simulink model "powertrain_model_simulink"  (R2023b)
settings: Solver=VariableStepAuto  StartTime=0.0  StopTime=20  RelTol=1e-3
undefined symbols (not defined in the file or in its folder): ts_equivalent_resistance
libraries: nesl_utility x9, fl_lib x7, ee_lib x7, simulink x1, batt_lib x1
settings Model: Creator=bglen  LastModifiedBy=bglen

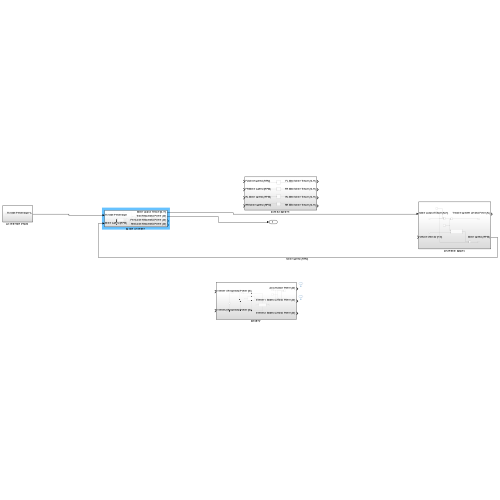
[thumbnail: Simulink's stored preview of the top-level diagram]
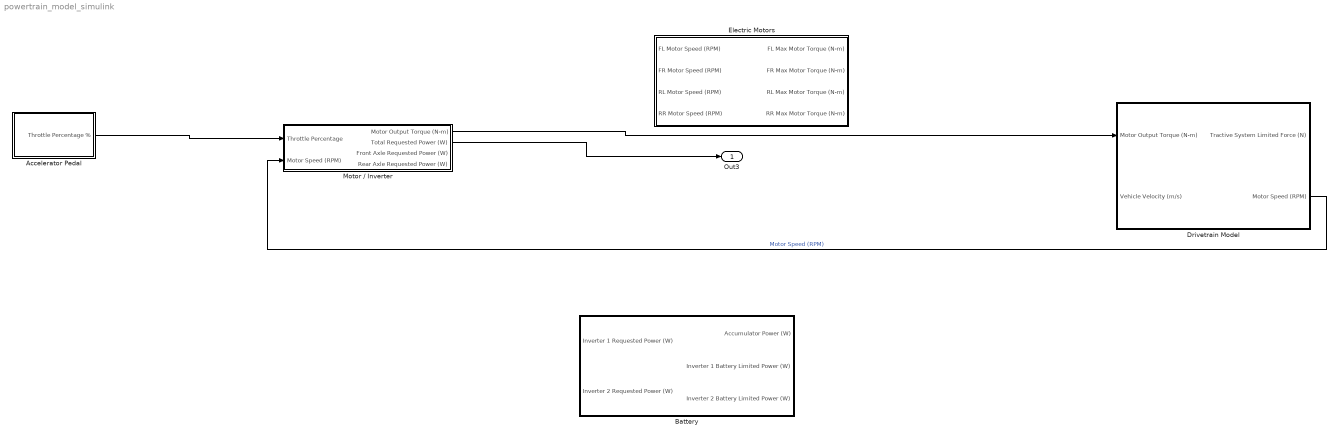
== system powertrain_model_simulink ==
  Accelerator Pedal : Subsystem
  Battery : Subsystem
  Drivetrain Model : Subsystem
  Electric Motors : Subsystem
  Motor / Inverter : Subsystem
  Out3 : Outport
  wires:
  Motor / Inverter/1(Motor Output Torque (N-m)) -> Drivetrain Model/1(Motor Output Torque (N-m))
  Motor / Inverter/2(Total Requested Power (W)) -> Out3/1
  Accelerator Pedal/1(Throttle Percentage %) -> Motor / Inverter/1(Throttle Percentage)
  Drivetrain Model/2(Motor Speed (RPM)) -> Motor / Inverter/2(Motor Speed (RPM))  "Motor Speed (RPM)"

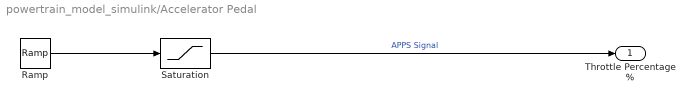
== system powertrain_model_simulink/Accelerator Pedal ==
  Ramp : simulink/Sources/Ramp  slope=4  start=0  InitialOutput=0
  Saturation : Saturate  UpperLimit=1  LowerLimit=0
  Throttle Percentage % : Outport
  wires:
  Saturation/1 -> Throttle Percentage %/1  "APPS Signal"
  Ramp/1 -> Saturation/1

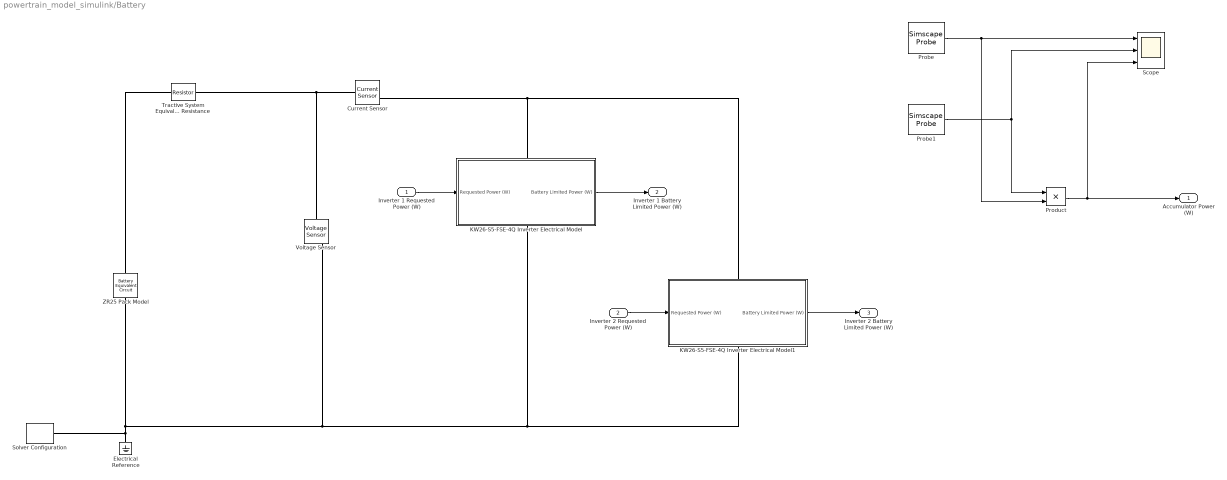
== system powertrain_model_simulink/Battery ==
  Inverter 1 Requested Power (W) : Inport
  Inverter 2 Requested Power (W) : Inport  Port=2
  Current Sensor : fl_lib/Electrical/Electrical Sensors/Current Sensor
  Electrical Reference : fl_lib/Electrical/Electrical Elements/Electrical Reference
  KW26-S5-FSE-4Q Inverter Electrical Model : Subsystem
      settings: PortSchema="{\"entries\":[{\"content\":{\"sides\":[{\"content\":{\"connectorIds\":[\"In1\"]},\"type\":\"ConnectorPlacement.EquallySpacedRectSide\",\"uuid\":\"23f200cd-6174-4ea5-b281-640ad05ed590\"},{\"content\":{\"connectorIds\":[\"Out1\"],\"side\":\"RIGHT\"},\"type\":\"ConnectorPlacement.EquallySpacedRectSide\",\"uuid\":\"19e54f00-a657-433d-b717-823657cd0153\"},{\"content\":{\"connectorIds\":[\"LConn1\"],\"side\":\"TOP\"},\"type\":\"ConnectorPlacement.EquallySpacedRectSide\",\"uuid\":\"a44b7635-6f3a-41c2-8d23-941c3ed86804\"},{\"content\":{\"connectorIds\":[\"RConn1\"],\"side\":\"BOTTOM\"},\"type\":\"ConnectorPlacement.EquallySpacedRectSide\",\"uuid\":\"02d96f81-f414-45e4-b3a2-9210237ffb13\"}]},\"type\":\"ConnectorPlacement.EquallySpacedConnector\",\"uuid\":\"152a73da-5f7e-4c02-a782-729b53bb1c10\"}],\"packageUris\":[\"http://schema.mathworks.com/mf0/Connector/R2020b\"],\"version\":\"1.0\"}"
  KW26-S5-FSE-4Q Inverter Electrical Model1 : Subsystem
      settings: PortSchema="{\"entries\":[{\"content\":{\"sides\":[{\"content\":{\"connectorIds\":[\"In1\"]},\"type\":\"ConnectorPlacement.EquallySpacedRectSide\",\"uuid\":\"23f200cd-6174-4ea5-b281-640ad05ed590\"},{\"content\":{\"connectorIds\":[\"Out1\"],\"side\":\"RIGHT\"},\"type\":\"ConnectorPlacement.EquallySpacedRectSide\",\"uuid\":\"19e54f00-a657-433d-b717-823657cd0153\"},{\"content\":{\"connectorIds\":[\"LConn1\"],\"side\":\"TOP\"},\"type\":\"ConnectorPlacement.EquallySpacedRectSide\",\"uuid\":\"a44b7635-6f3a-41c2-8d23-941c3ed86804\"},{\"content\":{\"connectorIds\":[\"RConn1\"],\"side\":\"BOTTOM\"},\"type\":\"ConnectorPlacement.EquallySpacedRectSide\",\"uuid\":\"02d96f81-f414-45e4-b3a2-9210237ffb13\"}]},\"type\":\"ConnectorPlacement.EquallySpacedConnector\",\"uuid\":\"152a73da-5f7e-4c02-a782-729b53bb1c10\"}],\"packageUris\":[\"http://schema.mathworks.com/mf0/Connector/R2020b\"],\"version\":\"1.0\"}"
  Probe : SimscapeProbe  BoundBlock=271  Variables={V}
  Probe1 : SimscapeProbe  BoundBlock=272  Variables={I}
  Product : Product
  Scope : Scope  NumInputPorts=3
  Solver Configuration : nesl_utility/Solver Configuration  PhysicalDomain=network_engine_domain  SubClassName=solver  LeftPortType=input  RightPortType=generic  Tones=[]  Harmonics=[]  SimulateNoise=off  Profile=off  UseLocalSampling=off  EnableSwitchedLinearOptims=on  FrequencyDomain=off  UseCCode=off  RelTol=0.001  AbsTol=0.001  MinStep=1e-09  ToWorkspace=off  RevertToSquareIcSolve=off  NumHomotopyIterations=100  PhasorMode=off  PhasorModeNumHarmonics=1  ConsistencySolver=NEWTON_XTOL_AFTER_FTOL  IndexReductionMethod=DerivativeReplacement  DoDC=off  ResidualTolerance=1e-09  ConsistencyTolSource=GLOBAL  ConsistencyAbsTol=0.001  ConsistencyRelTol=0.001  ConsistencyTolFactor=0.001  UseLocalSolver=off  LocalSolverChoice=NE_BACKWARD_EULER_ADVANCER  ResolveIndetEquations=on  FunctionEvalNumThread=1  LocalSolverSampleTime=0.001  DoFixedCost=off  MaxNonlinIter=3  MaxModeIter=2  ComputeImpulses=off  ImpulseIterations=2  LinearAlgebra=auto  LinearAlgebraNumThread=0  EquationFormulation=NE_TIME_EF  DelaysMemoryBudget=1024  AutomaticFiltering=on  FilteringTimeConstant=0.001  PartitionStorageMethod=AS_NEEDED  PartitionMemoryBudget=1024  PartitionMethod=ROBUST  MultibodyUseLocalSolver=off  MultibodyLocalSolverChoice=ODE1  MultibodyLocalSolverSampleTime=0.001
  Tractive System Equivalent Resistance : ee_lib/Passive/Resistor  R=ts_equivalent_resistance Ohm  enable_R_tol=ee.enum.toleranceApplication.none  R_tol=5  tol_distribution=ee.enum.toleranceDistribution.uniform  nSigma=4  enable_operating_limits=ee.enum.enable.no  operating_limit_action=ee.enum.passive.reportOpLim.warn  power_rating=1 W  max_working_voltage=100 V  enable_faults=ee.enum.enable.no  fault_action=simscape.enum.assert.action.none  R_faulted=inf Ohm  fault_trigger=ee.enum.faults.faultTrigger.temporal  t_fault=1 s  max_permissible_current=1 A  t_fail_on_current=1 s  noise_mode=ee.enum.sources.noise.Disabled  Tdevice=25 degC  sample_time=1e-3 s  repeatability=ee.enum.ic.repeatability.notRepeatable  user_seed=0  auto_seed=3499211588  faulted_specify=off  faulted_priority=None  faulted=0  power_derating_T1=70 degC  power_derating_T2=155 degC  operating_temperature_range_vec=[-50, 150] degC  alpha=3.93e-3 1/K  Tmeas=25 degC  thermal_mass=100 J/K  temperature_specify=off  temperature_priority=High  temperature=298.15 K  temperature_nominal_specify=off  temperature_nominal_unit=K  temperature_nominal_value=1
  Voltage Sensor : fl_lib/Electrical/Electrical Sensors/Voltage Sensor
  ZR25 Pack Model : batt_lib/Cells/Battery Equivalent Circuit  BatteryCapacity=pack_nominal_capacity A*hr  ThermalModel=simscape.battery.enum.cells.BatteryThermalModel.ConstantTemperature  ExtrapolationMethod=simscape.enum.extrapolation.nearest  EnableFaultExotherm=false  TriggerTemperature=350 K  SOCBreakpoints=pack_SOC  TemperatureBreakpoints=pack_temps degC  OpenCircuitVoltage=[3.5057, 3.566, 3.6337, 3.7127, 3.9259, 4.0777, 4.1928] V  OpenCircuitVoltageThermal=pack_OCV V  VoltageRange=[0, inf] V  HysteresisModel=simscape.battery.enum.cells.HysteresisModel.none  MaximumHysteresisVoltage=[0, 0, 0, 0, 0, 0, 0] V  InstantaneousHysteresisVoltage=[0, 0, 0, 0, 0, 0, 0] V  HysteresisRate=0.1  MaximumHysteresisVoltageThermal=[0, 0, 0; 0, 0, 0; 0, 0, 0; 0, 0, 0; 0, 0, 0; 0, 0, 0; 0, 0, 0] V  InstantaneousHysteresisVoltageThermal=[0, 0, 0; 0, 0, 0; 0, 0, 0; 0, 0, 0; 0, 0, 0; 0, 0, 0; 0, 0, 0] V  HysteresisRateThermal=0.1  ResistanceSOCBreakpoints=pack_SOC  ResistanceTemperatureBreakpoints=pack_temps degC  CurrentDirectionality=simscape.battery.enum.cells.BatteryEnable.Disabled  R0=[.0085, .0085, .0087, .0082, .0083, .0085, .0085] Ohm  R0Thermal=pack_DC_IR Ohm  DischargeR0=[.0085, .0085, .0087, .0082, .0083, .0085, .0085] Ohm  ChargeR0=[.0085, .0085, .0087, .0082, .0083, .0085, .0085] Ohm  ChargeR0Thermal=[.0117, .0085, .009; .011, .0085, .009; .0114, .0087, .0092; .0107, .0082, .0088; .0107, .0083, .0091; .0113, .0085, .0089; .0116, .0085, .0089] Ohm  DischargeR0Thermal=[.0117, .0085, .009; .011, .0085, .009; .0114, .0087, .0092; .0107, .0082, .0088; .0107, .0083, .0091; .0113, .0085, .0089; .0116, .0085, .0089] Ohm  SelfDischargeResistor=simscape.battery.enum.cells.BatteryEnable.Disabled  SelfDischargeR=7e3 Ohm  SelfDischargeRThermal=[8000, 7000, 6000] Ohm  RCPairs=simscape.battery.enum.cells.RCPairs.noDynamics  R1=[.0029, .0024, .0026, .0016, .0023, .0018, .0017] Ohm  Tau1=[36, 45, 105, 29, 77, 33, 39] s  R2=[.0029, .0024, .0026, .0016, .0023, .0018, .0017] Ohm  Tau2=[36, 45, 105, 29, 77, 33, 39] s  R3=[.0029, .0024, .0026, .0016, .0023, .0018, .0017] Ohm  Tau3=[36, 45, 105, 29, 77, 33, 39] s  DischargeR1=[.0029, .0024, .0026, .0016, .0023, .0018, .0017] Ohm  DischargeTau1=[36, 45, 105, 29, 77, 33, 39] s  ChargeR1=[.0029, .0024, .0026, .0016, .0023, .0018, .0017] Ohm  ChargeTau1=[36, 45, 105, 29, 77, 33, 39] s  DischargeR2=[.0029, .0024, .0026, .0016, .0023, .0018, .0017] Ohm  DischargeTau2=[36, 45, 105, 29, 77, 33, 39] s  ChargeR2=[.0029, .0024, .0026, .0016, .0023, .0018, .0017] Ohm  ChargeTau2=[36, 45, 105, 29, 77, 33, 39] s  DischargeR3=[.0029, .0024, .0026, .0016, .0023, .0018, .0017] Ohm  DischargeTau3=[36, 45, 105, 29, 77, 33, 39] s  ChargeR3=[.0029, .0024, .0026, .0016, .0023, .0018, .0017] Ohm  ChargeTau3=[36, 45, 105, 29, 77, 33, 39] s  R1Thermal=[.0109, .0029, .0013; .0069, .0024, .0012; .0047, .0026, .0013; .0034, .0016, .001; .0033, .0023, .0014; .0033, .0018, .0011; .0028, .0017, .0011] Ohm  Tau1Thermal=[20, 36, 39; 31, 45, 39; 109, 105, 61; 36, 29, 26; 59, 77, 67; 40, 33, 29; 25, 39, 33] s  R2Thermal=[.0109, .0029, .0013; .0069, .0024, .0012; .0047, .0026, .0013; .0034, .0016, .001; .0033, .0023, .0014; .0033, .0018, .0011; .0028, .0017, .0011] Ohm  Tau2Thermal=[20, 36, 39; 31, 45, 39; 109, 105, 61; 36, 29, 26; 59, 77, 67; 40, 33, 29; 25, 39, 33] s  R3Thermal=[.0109, .0029, .0013; .0069, .0024, .0012; .0047, .0026, .0013; .0034, .0016, .001; .0033, .0023, .0014; .0033, .0018, .0011; .0028, .0017, .0011] Ohm  Tau3Thermal=[20, 36, 39; 31, 45, 39; 109, 105, 61; 36, 29, 26; 59, 77, 67; 40, 33, 29; 25, 39, 33] s  DischargeR1Thermal=[.0109, .0029, .0013; .0069, .0024, .0012; .0047, .0026, .0013; .0034, .0016, .001; .0033, .0023, .0014; .0033, .0018, .0011; .0028, .0017, .0011] Ohm  DischargeTau1Thermal=[20, 36, 39; 31, 45, 39; 109, 105, 61; 36, 29, 26; 59, 77, 67; 40, 33, 29; 25, 39, 33] s  ChargeR1Thermal=[.0109, .0029, .0013; .0069, .0024, .0012; .0047, .0026, .0013; .0034, .0016, .001; .0033, .0023, .0014; .0033, .0018, .0011; .0028, .0017, .0011] Ohm  ChargeTau1Thermal=[20, 36, 39; 31, 45, 39; 109, 105, 61; 36, 29, 26; 59, 77, 67; 40, 33, 29; 25, 39, 33] s  DischargeR2Thermal=[.0109, .0029, .0013; .0069, .0024, .0012; .0047, .0026, .0013; .0034, .0016, .001; .0033, .0023, .0014; .0033, .0018, .0011; .0028, .0017, .0011] Ohm  DischargeTau2Thermal=[20, 36, 39; 31, 45, 39; 109, 105, 61; 36, 29, 26; 59, 77, 67; 40, 33, 29; 25, 39, 33] s  ChargeR2Thermal=[.0109, .0029, .0013; .0069, .0024, .0012; .0047, .0026, .0013; .0034, .0016, .001; .0033, .0023, .0014; .0033, .0018, .0011; .0028, .0017, .0011] Ohm  ChargeTau2Thermal=[20, 36, 39; 31, 45, 39; 109, 105, 61; 36, 29, 26; 59, 77, 67; 40, 33, 29; 25, 39, 33] s  DischargeR3Thermal=[.0109, .0029, .0013; .0069, .0024, .0012; .0047, .0026, .0013; .0034, .0016, .001; .0033, .0023, .0014; .0033, .0018, .0011; .0028, .0017, .0011] Ohm  DischargeTau3Thermal=[20, 36, 39; 31, 45, 39; 109, 105, 61; 36, 29, 26; 59, 77, 67; 40, 33, 29; 25, 39, 33] s  ChargeR3Thermal=[.0109, .0029, .0013; .0069, .0024, .0012; .0047, .0026, .0013; .0034, .0016, .001; .0033, .0023, .0014; .0033, .0018, .0011; .0028, .0017, .0011] Ohm  ChargeTau3Thermal=[20, 36, 39; 31, 45, 39; 109, 105, 61; 36, 29, 26; 59, 77, 67; 40, 33, 29; 25, 39, 33] s  CyclingAgingMethod=simscape.battery.enum.cells.CyclingAgingMethod.disabled  NumDisCycles=100  OCVChange=0  R0Change=0  CapacityChange=0  SelfDischargeRChange=0  R1Change=0  R2Change=0  R3Change=0  NumDisCyclesBreakpoints=[0, 100, 200, 300]  AgingTemperatureBreakpoints=[298.15, 323.15] K  OCVChangeVec=[0, 0, 0, 0]  R0ChangeVec=[0, 0, 0, 0]  CapacityChangeVec=[0, 0, 0, 0]  SelfDischargeRChangeVec=[0, 0, 0, 0]  R1ChangeVec=[0, 0, 0, 0]  R2ChangeVec=[0, 0, 0, 0]  R3ChangeVec=[0, 0, 0, 0]  OCVChangeThermal=[0, 0; 0, 0; 0, 0; 0, 0]  R0ChangeThermal=[0, 0; 0, 0; 0, 0; 0, 0]  CapacityChangeThermal=[0, 0; 0, 0; 0, 0; 0, 0]  SelfDischargeRChangeThermal=[0, 0; 0, 0; 0, 0; 0, 0]  R1ChangeThermal=[0, 0; 0, 0; 0, 0; 0, 0]  R2ChangeThermal=[0, 0; 0, 0; 0, 0; 0, 0]  R3ChangeThermal=[0, 0; 0, 0; 0, 0; 0, 0]  CalendarAgeResistance=simscape.battery.enum.cells.BatteryEnable.Disabled  CalendarAgeCapacity=simscape.battery.enum.cells.BatteryEnable.Disabled  CalendarAgingMethod=simscape.battery.enum.cells.CalendarAgingMethod.equation  StorageVariable=simscape.battery.enum.cells.StorageVariable.OCV  OCVDuringStorage=0.9  SOCDuringStorage=0.6  StorageTimeIntervals=[0] d  StorageTemperatures=[273] K  ResistanceScalingOCV=2.2134e6  ResistanceScalingOCVOffset=1.632e6  ResistanceExponentialIncrease=0.515833569 V  ResistanceTimeExponent=0.75  ResistanceAgeTemperatureBreakpoints=[273.15, 298.15, 323.15] K  ResistanceAgeTimeBreakpoints=[0, 90, 180, 270] d  PercentResistanceChange=[0, 0, 0]  ResistanceTimeBreakpoints=100 d  PercentResistanceChangeThermal=[0, 0, 0; 0, 0, 0; 0, 0, 0; 0, 0, 0]  CapacityScalingOCV=1.5097e07  CapacityScalingOCVOffset=8.3625e06  CapacityExponentialIncrease=0.6011 V  CapacityTimeExponent=0.75  CapacityAgeTemperatureBreakpoints=[273.15, 298.15, 323.15] K  CapacityAgeTimeBreakpoints=[0, 90, 180, 270] d  PercentCapacityChange=[0, 0, 0]  CapacityTimeBreakpoints=100 d  PercentCapacityChangeThermal=[0, 0, 0; 0, 0, 0; 0, 0, 0; 0, 0, 0]  SimulationTemperature=298.15 degC  BatteryThermalMass=100 J/K  ReversibleHeatModel=simscape.battery.enum.cells.ReversibleHeatModel.Disabled  EntropicCoefficient=[0, 0, 0, 0, 0, 0, 0] mV/K  AddedResistance=1e5 Ohm  ShortedResistance=1e-6 Ohm  ExothermModel=simscape.battery.enum.cells.ExothermModel.analytical  TabulateWithSOC=false  SOCvecExotherm=[0, .5, 1]  CurrInterruptTempSOC=[420, 420, 420] K  TotalHeatOfReactionSOC=[23000, 23000, 23000] J  CurrentInterruptTemperature=420 K  TotalHeatOfReaction=23e3 J  ExothermOnsetTemperature=350 K  ExothermOnsetTempSOC=[350, 350, 350] K  OnsetTempRate=0.02 K/min  ActivationEnergy=160e3 J/mol  ActivationEnergySOC=[160000, 160000, 160000] J/mol  ReactionOrder=1  ReactionOrderSOC=[1, 1, 1]  TemperaturesFromARC=[323, 373, 423, 438, 463, 483, 513, 543, 545, 547, 549, 551, 553, 573, 623, 773, 923, 943, 1003, 1063, 1113, 1123, 1133, 1153, 1173] K  TemperatureRatesFromARC=[.0001, .001, .025, .2, .4, .6, 1.1, 1.3, 1.9, 3, 5, 11.6, 183.3, 191.6, 200, 208.3, 200, 175, 8.33, 1.33, .33, .2, .13, .0017, .00017] K/s  TempRateVecARCSOC=repmat([.0001, .001, .025, .2, .4, .6, 1.1, 1.3, 1.9, 3, 5, 11.6, 183.3, 191.6, 200, 208.3, 200, 175, 8.33, 1.33, .33, .2, .13, .0017, .00017]', 1, 3) K/s  PercentThermalMassVented=40  PercentThermalMassVentedSOC=[40, 40, 40]  EnableFaultAddRes=false  EnableFaultShort=false  faultTriggerType=simscape.fault.triggertype.external  stateOfCharge_specify=on  stateOfCharge_priority=High  stateOfCharge=1  stateOfCharge_nominal_specify=off  stateOfCharge_nominal_unit=1  stateOfCharge_nominal_value=1  numCycles_specify=off  numCycles_priority=High  numCycles=0  numCycles_nominal_specify=off  numCycles_nominal_unit=1  numCycles_nominal_value=1  batteryVoltage_specify=off  batteryVoltage_priority=None  batteryVoltage=0 V  batteryVoltage_nominal_specify=off  batteryVoltage_nominal_unit=V  batteryVoltage_nominal_value=3.73  batteryCurrent_specify=off  batteryCurrent_priority=None  batteryCurrent=0 A  batteryCurrent_nominal_specify=off  batteryCurrent_nominal_unit=A  batteryCurrent_nominal_value=1  batteryTemperature_specify=off  batteryTemperature_priority=High  batteryTemperature=298.15 K  batteryTemperature_nominal_specify=off  batteryTemperature_nominal_unit=K  batteryTemperature_nominal_value=1  hysteresisState_specify=off  hysteresisState_priority=High  hysteresisState=0  hysteresisState_nominal_specify=off  hysteresisState_nominal_unit=1  hysteresisState_nominal_value=1  isExothermFaulted_specify=off  isExothermFaulted_priority=None  isExothermFaulted=0  isExothermFaulted_nominal_specify=off  isExothermFaulted_nominal_unit=1  isExothermFaulted_nominal_value=1  isCurrentInterruptionTempExceeded_specify=off  isCurrentInterruptionTempExceeded_priority=None  isCurrentInterruptionTempExceeded=0  isCurrentInterruptionTempExceeded_nominal_specify=off  isCurrentInterruptionTempExceeded_nominal_unit=1  isCurrentInterruptionTempExceeded_nominal_value=1  reactionHeatRate_specify=off  reactionHeatRate_priority=None  reactionHeatRate=0 W  reactionHeatRate_nominal_specify=off  reactionHeatRate_nominal_unit=W  reactionHeatRate_nominal_value=1  reactionExtent_specify=off  reactionExtent_priority=None  reactionExtent=0  reactionExtent_nominal_specify=off  reactionExtent_nominal_unit=1  reactionExtent_nominal_value=1
      settings: InternalSimscapePortConfiguration="{\"Bottom\":[],\"Left\":[{\"id\":\"p\",\"label\":\"+\",\"type\":\"foundation.electrical.electrical\"}],\"Right\":[{\"id\":\"n\",\"label\":\"-\",\"type\":\"foundation.electrical.electrical\"}],\"Top\":[]}"
  Accumulator Power (W) : Outport
  Inverter 1 Battery Limited Power (W) : Outport  Port=2
  Inverter 2 Battery Limited Power (W) : Outport  Port=3
  wires:
  Probe/1 -> Scope/1, Product/2
  Probe1/1 -> Scope/2, Product/1
  Product/1 -> Accumulator Power (W)/1, Scope/3
  Inverter 1 Requested Power (W)/1 -> KW26-S5-FSE-4Q Inverter Electrical Model/1(Requested Power (W))
  KW26-S5-FSE-4Q Inverter Electrical Model/1(Battery Limited Power (W)) -> Inverter 1 Battery Limited Power (W)/1
  KW26-S5-FSE-4Q Inverter Electrical Model1/1(Battery Limited Power (W)) -> Inverter 2 Battery Limited Power (W)/1
  Inverter 2 Requested Power (W)/1 -> KW26-S5-FSE-4Q Inverter Electrical Model1/1(Requested Power (W))
  connections:
  Electrical Reference/LConn1 -- KW26-S5-FSE-4Q Inverter Electrical Model1/RConn1 -- KW26-S5-FSE-4Q Inverter Electrical Model/RConn1 -- Voltage Sensor/RConn2 -- ZR25 Pack Model/RConn1 -- Solver Configuration/RConn1
  Tractive System Equivalent Resistance/RConn1 -- Current Sensor/LConn1 -- Voltage Sensor/LConn1
  Current Sensor/RConn2 -- KW26-S5-FSE-4Q Inverter Electrical Model1/LConn1 -- KW26-S5-FSE-4Q Inverter Electrical Model/LConn1
  Tractive System Equivalent Resistance/LConn1 -- ZR25 Pack Model/LConn1

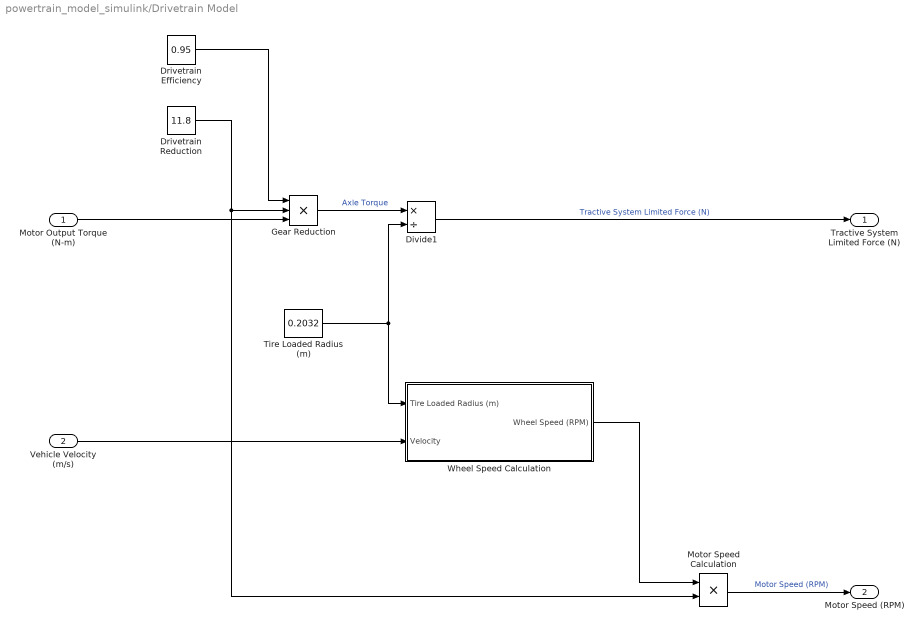
== system powertrain_model_simulink/Drivetrain Model ==
  Motor Output Torque (N-m) : Inport
  Vehicle Velocity (m/s) : Inport  Port=2
  "  Motor Speed Calculation" : Product
  Divide1 : Product  Inputs=*/
  Drivetrain Efficiency : Constant  Value=0.95
  Drivetrain Reduction : Constant  Value=11.8
  Gear Reduction : Product  Inputs=3
  Tire Loaded Radius (m) : Constant  Value=0.2032
  Wheel Speed Calculation : Subsystem
  Tractive System Limited Force (N) : Outport
  Motor Speed (RPM) : Outport  Port=2
  wires:
  Divide1/1 -> Tractive System Limited Force (N)/1  "Tractive System Limited Force (N)"
  Tire Loaded Radius (m)/1 -> Wheel Speed Calculation/1(Tire Loaded Radius (m)), Divide1/2
  Gear Reduction/1 -> Divide1/1  "Axle Torque"
  Motor Output Torque (N-m)/1 -> Gear Reduction/3
  Drivetrain Efficiency/1 -> Gear Reduction/1
  Drivetrain Reduction/1 -> "  Motor Speed Calculation"/2, Gear Reduction/2
  Vehicle Velocity (m/s)/1 -> Wheel Speed Calculation/2(Velocity)
  Wheel Speed Calculation/1(Wheel Speed (RPM)) -> "  Motor Speed Calculation"/1
  "  Motor Speed Calculation"/1 -> Motor Speed (RPM)/1  "Motor Speed (RPM)"

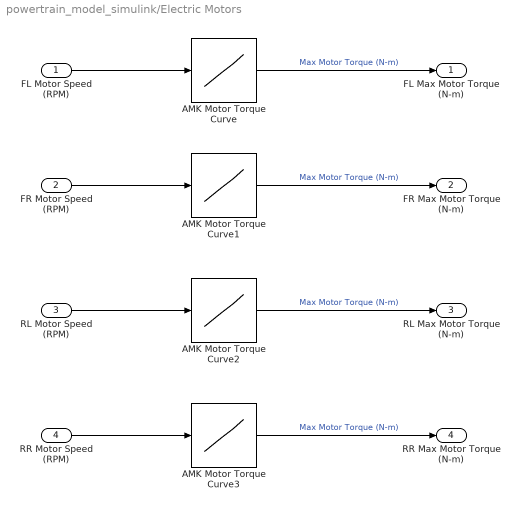
== system powertrain_model_simulink/Electric Motors ==
  FL Motor Speed (RPM) : Inport
  FR Motor Speed (RPM) : Inport  Port=2
  RL Motor Speed (RPM) : Inport  Port=3
  RR Motor Speed (RPM) : Inport  Port=4
  AMK Motor Torque Curve{,1..3} (4 alike) : Lookup_n-D  NumberOfTableDimensions=1  BreakpointsForDimension1=[0;28.3870968;1447.74194;3179.35484;4740.64516;7267.09677;9055.48387;10872.2581;12178.0645;13029.6774;13994.8387;14846.4516;15612.9032;16095.4839;16805.1613;17571.6129;18423.2258;19274.8387;19785.8065;19984.5161]  Table=[21.31;21.3068182;21.3068182;21.3068182;21.3068182;21.3068182;21.3068182;21.3068182;21.3068182;21.3068182;21.3068182;21.3068182;21.3068182;20.9659091;19.9431818;18.5795455;17.0454545;15.3409091;14.1477273;13.6363636]  InternalRulePriority=Speed  RndMeth=Simplest
  FL Max Motor Torque (N-m) : Outport
  FR Max Motor Torque (N-m) : Outport  Port=2
  RL Max Motor Torque (N-m) : Outport  Port=3
  RR Max Motor Torque (N-m) : Outport  Port=4
  wires:
  AMK Motor Torque Curve/1 -> FL Max Motor Torque (N-m)/1  "Max Motor Torque (N-m)"
  FL Motor Speed (RPM)/1 -> AMK Motor Torque Curve/1
  FR Motor Speed (RPM)/1 -> AMK Motor Torque Curve1/1
  AMK Motor Torque Curve1/1 -> FR Max Motor Torque (N-m)/1  "Max Motor Torque (N-m)"
  RL Motor Speed (RPM)/1 -> AMK Motor Torque Curve2/1
  AMK Motor Torque Curve2/1 -> RL Max Motor Torque (N-m)/1  "Max Motor Torque (N-m)"
  RR Motor Speed (RPM)/1 -> AMK Motor Torque Curve3/1
  AMK Motor Torque Curve3/1 -> RR Max Motor Torque (N-m)/1  "Max Motor Torque (N-m)"

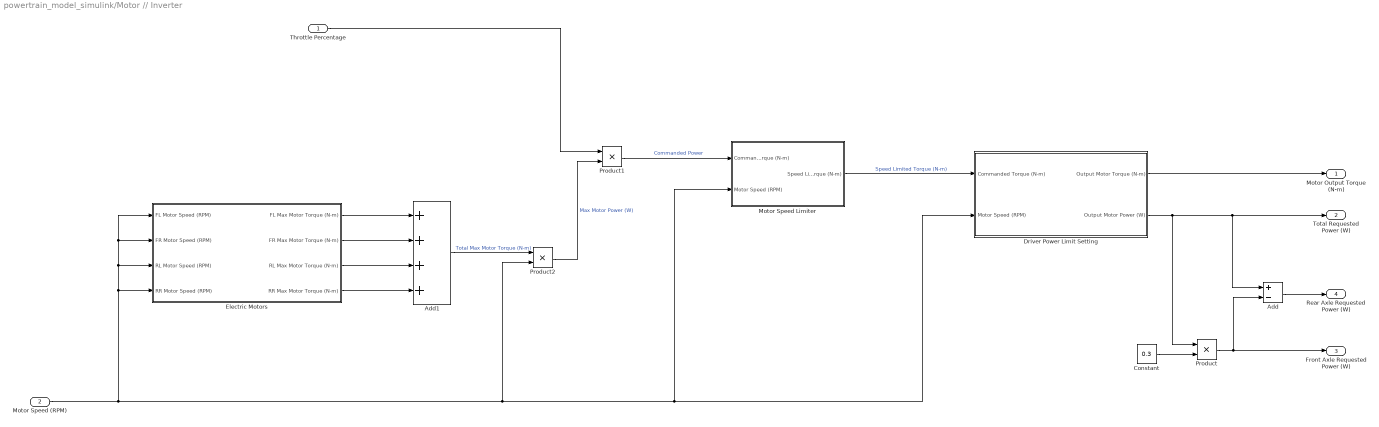
== system powertrain_model_simulink/Motor // Inverter ==
  Throttle Percentage : Inport
  Motor Speed (RPM) : Inport  Port=2
  Add : Sum  Inputs=+-
  Add1 : Sum  Inputs=++++
  Constant : Constant  Value=0.3
  Driver Power Limit Setting : Subsystem
  Electric Motors : Subsystem
  Motor Speed Limiter : Subsystem
  Product : Product
  Product1 : Product
  Product2 : Product
  Motor Output Torque (N-m) : Outport
  Total Requested Power (W) : Outport  Port=2
  Front Axle Requested Power (W) : Outport  Port=3
  Rear Axle Requested Power (W) : Outport  Port=4
  wires:
  Throttle Percentage/1 -> Product1/1
  Product1/1 -> Motor Speed Limiter/1(Commanded Torque (N-m))  "Commanded Power"
  Motor Speed (RPM)/1 -> Electric Motors/1(FL Motor Speed (RPM)), Electric Motors/2(FR Motor Speed (RPM)), Electric Motors/3(RL Motor Speed (RPM)), Electric Motors/4(RR Motor Speed (RPM)), Product2/2, Motor Speed Limiter/2(Motor Speed (RPM)), Driver Power Limit Setting/2(Motor Speed (RPM))
  Motor Speed Limiter/1(Speed Limited Motor Torque (N-m)) -> Driver Power Limit Setting/1(Commanded Torque (N-m))  "Speed Limited Torque (N-m)"
  Driver Power Limit Setting/1(Output Motor Torque (N-m)) -> Motor Output Torque (N-m)/1
  Driver Power Limit Setting/2(Output Motor Power (W)) -> Total Requested Power (W)/1, Add/1, Product/1
  Constant/1 -> Product/2
  Product/1 -> Front Axle Requested Power (W)/1, Add/2
  Add/1 -> Rear Axle Requested Power (W)/1
  Electric Motors/1(FL Max Motor Torque (N-m)) -> Add1/1
  Electric Motors/2(FR Max Motor Torque (N-m)) -> Add1/2
  Electric Motors/3(RL Max Motor Torque (N-m)) -> Add1/3
  Electric Motors/4(RR Max Motor Torque (N-m)) -> Add1/4
  Add1/1 -> Product2/1  "Total Max Motor Torque (N-m)"
  Product2/1 -> Product1/2  "Max Motor Power (W)"

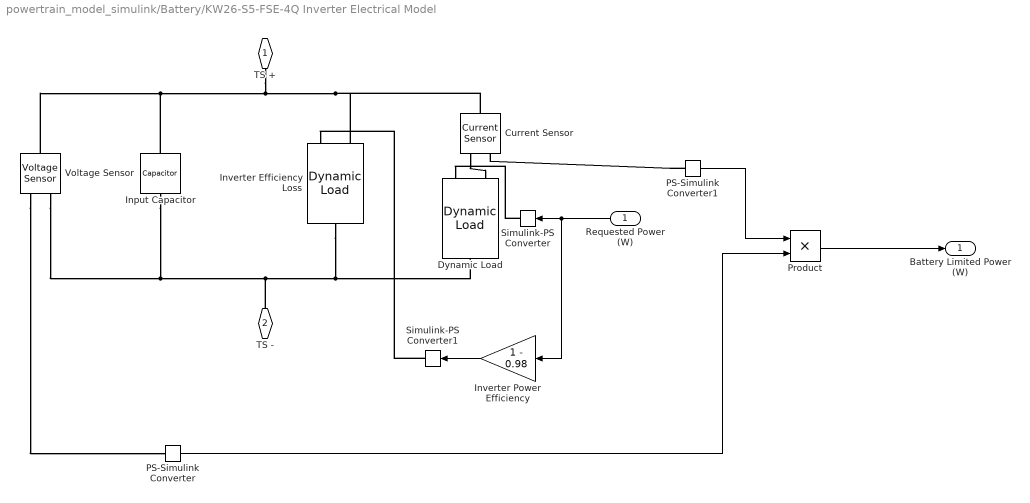
== system powertrain_model_simulink/Battery/KW26-S5-FSE-4Q Inverter Electrical Model ==
  Requested Power (W) : Inport
  Current Sensor : fl_lib/Electrical/Electrical Sensors/Current Sensor
  Dynamic Load : ee_lib/Passive/Dynamic Load  load_type=ee.enum.dc_ac.dc  min_supply_voltage=250 V  pow_min=1e-3 W  G_reverse=1e-6 S  deltaV=1e-3 V  f0=60 Hz  Vrms_min=200 V  Pmin=1e-3 W  enable_fault=simscape.enum.onoff.off  fault_action=simscape.enum.assert.action.none  t_fault=1 s  open_conductance=1e-4 S
      settings: InternalSimscapePortConfiguration="{\"Bottom\":[],\"Left\":[{\"id\":\"p\",\"label\":\"+\",\"type\":\"foundation.electrical.electrical\"}],\"Right\":[{\"id\":\"n\",\"label\":\"-\",\"type\":\"foundation.electrical.electrical\"}],\"Top\":[{\"id\":\"P\",\"label\":\"P\",\"type\":\"input\"}]}"
  Input Capacitor : ee_lib/Passive/Capacitor  cap_option=ee.enum.passive.capacitor.capOption.const  c=150 uF  Cvec=[1e-05, 1e-06] F  Vvec=[0, 10] V  CV_table_symmetry=ee.enum.passive.capacitor.tableSymmetry.yes  f_vec=[1, 10] kHz  DFext_vec=[.8, 1.2]  enable_C_tol=ee.enum.toleranceApplication.none  averaging_period=0 s  C_tol=5  tol_distribution=ee.enum.toleranceDistribution.uniform  nSigma=4  r=1e-6 Ohm  g=0 1/Ohm  enable_operating_limits=ee.enum.enable.no  operating_limit_action=ee.enum.passive.reportOpLim.warn  max_working_voltage_range=[-25, 25] V  power_rating=1 W  enable_faults=ee.enum.enable.no  fault_action=simscape.enum.assert.action.none  Cscale_faulted=100  R_faulted=1e-3 Ohm  G_faulted=0 1/Ohm  tau_fault=1e-3 s  fault_trigger=ee.enum.faults.faultTrigger.temporal  t_fault=1 s  max_permissible_voltage_range=[-100, 100] V  t_fail_on_voltage=1 s  i_specify=off  i_priority=None  i=0 A  i_nominal_specify=off  i_nominal_unit=A  i_nominal_value=1  v_specify=off  v_priority=None  v=0 V  v_nominal_specify=off  v_nominal_unit=V  v_nominal_value=1  vc_specify=off  vc_priority=High  vc=0 V  vc_nominal_specify=off  vc_nominal_unit=V  vc_nominal_value=1
  Inverter Efficiency Loss : ee_lib/Passive/Dynamic Load  load_type=ee.enum.dc_ac.dc  min_supply_voltage=1 V  pow_min=1e-3 W  G_reverse=1e-6 S  deltaV=1e-3 V  f0=60 Hz  Vrms_min=200 V  Pmin=1e-3 W  enable_fault=simscape.enum.onoff.off  fault_action=simscape.enum.assert.action.none  t_fault=1 s  open_conductance=1e-4 S
      settings: InternalSimscapePortConfiguration="{\"Bottom\":[],\"Left\":[{\"id\":\"p\",\"label\":\"+\",\"type\":\"foundation.electrical.electrical\"}],\"Right\":[{\"id\":\"n\",\"label\":\"-\",\"type\":\"foundation.electrical.electrical\"}],\"Top\":[{\"id\":\"P\",\"label\":\"P\",\"type\":\"input\"}]}"
  Inverter Power Efficiency : Gain  Gain=1 - 0.98
  PS-Simulink Converter : nesl_utility/PS-Simulink Converter  PhysicalDomain=network_engine_domain  SubClassName=ps_output  LeftPortType=input  RightPortType=output  PseudoPeriodic=off  Frequencies=[]  VectorFormat=inherit  Unit=inherit  AffineConversion=off
  PS-Simulink Converter1 : nesl_utility/PS-Simulink Converter  PhysicalDomain=network_engine_domain  SubClassName=ps_output  LeftPortType=input  RightPortType=output  PseudoPeriodic=off  Frequencies=[]  VectorFormat=inherit  Unit=inherit  AffineConversion=off
  Product : Product
  Simulink-PS Converter : nesl_utility/Simulink-PS Converter  PhysicalDomain=network_engine_domain  SubClassName=ps_input  LeftPortType=input  RightPortType=output  PseudoPeriodic=off  Frequencies=[]  NoiseDistribution=none  NoiseParameters=[]  Unit=1  AffineConversion=off  FilteringAndDerivatives=provide  SimscapeFilterOrder=1  InputFilterTimeConstant=0.001  UdotUserProvided=0
  Simulink-PS Converter1 : nesl_utility/Simulink-PS Converter  PhysicalDomain=network_engine_domain  SubClassName=ps_input  LeftPortType=input  RightPortType=output  PseudoPeriodic=off  Frequencies=[]  NoiseDistribution=none  NoiseParameters=[]  Unit=1  AffineConversion=off  FilteringAndDerivatives=provide  SimscapeFilterOrder=1  InputFilterTimeConstant=0.001  UdotUserProvided=0
  Voltage Sensor : fl_lib/Electrical/Electrical Sensors/Voltage Sensor
  TS + : PMIOPort  Side=Left
  TS - : PMIOPort  Port=2  Side=Right
  Battery Limited Power (W) : Outport
  wires:
  Requested Power (W)/1 -> Inverter Power Efficiency/1, Simulink-PS Converter/1
  PS-Simulink Converter1/1 -> Product/1
  PS-Simulink Converter/1 -> Product/2
  Inverter Power Efficiency/1 -> Simulink-PS Converter1/1
  Product/1 -> Battery Limited Power (W)/1
  connections:
  Input Capacitor/RConn1 -- Inverter Efficiency Loss/RConn1 -- Dynamic Load/RConn1 -- TS -/RConn1 -- Voltage Sensor/RConn2
  Input Capacitor/LConn1 -- Current Sensor/LConn1 -- Inverter Efficiency Loss/LConn1 -- TS +/RConn1 -- Voltage Sensor/LConn1
  Simulink-PS Converter/RConn1 -- Dynamic Load/LConn2
  Voltage Sensor/RConn1 -- PS-Simulink Converter/LConn1
  Current Sensor/RConn2 -- Dynamic Load/LConn1
  PS-Simulink Converter1/LConn1 -- Current Sensor/RConn1
  Simulink-PS Converter1/RConn1 -- Inverter Efficiency Loss/LConn2

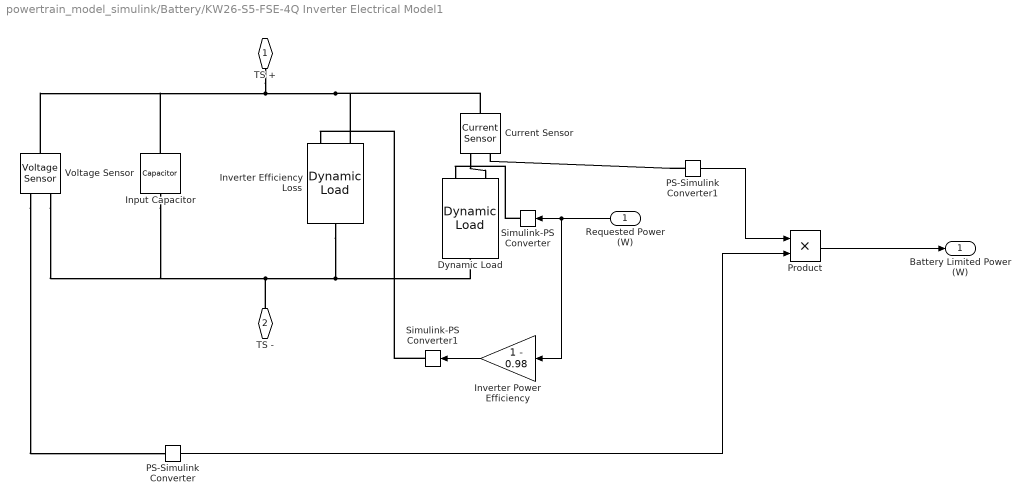
== system powertrain_model_simulink/Battery/KW26-S5-FSE-4Q Inverter Electrical Model1 ==
  Requested Power (W) : Inport
  Current Sensor : fl_lib/Electrical/Electrical Sensors/Current Sensor
  Dynamic Load : ee_lib/Passive/Dynamic Load  load_type=ee.enum.dc_ac.dc  min_supply_voltage=250 V  pow_min=1e-3 W  G_reverse=1e-6 S  deltaV=1e-3 V  f0=60 Hz  Vrms_min=200 V  Pmin=1e-3 W  enable_fault=simscape.enum.onoff.off  fault_action=simscape.enum.assert.action.none  t_fault=1 s  open_conductance=1e-4 S
      settings: InternalSimscapePortConfiguration="{\"Bottom\":[],\"Left\":[{\"id\":\"p\",\"label\":\"+\",\"type\":\"foundation.electrical.electrical\"}],\"Right\":[{\"id\":\"n\",\"label\":\"-\",\"type\":\"foundation.electrical.electrical\"}],\"Top\":[{\"id\":\"P\",\"label\":\"P\",\"type\":\"input\"}]}"
  Input Capacitor : ee_lib/Passive/Capacitor  cap_option=ee.enum.passive.capacitor.capOption.const  c=150 uF  Cvec=[1e-05, 1e-06] F  Vvec=[0, 10] V  CV_table_symmetry=ee.enum.passive.capacitor.tableSymmetry.yes  f_vec=[1, 10] kHz  DFext_vec=[.8, 1.2]  enable_C_tol=ee.enum.toleranceApplication.none  averaging_period=0 s  C_tol=5  tol_distribution=ee.enum.toleranceDistribution.uniform  nSigma=4  r=1e-6 Ohm  g=0 1/Ohm  enable_operating_limits=ee.enum.enable.no  operating_limit_action=ee.enum.passive.reportOpLim.warn  max_working_voltage_range=[-25, 25] V  power_rating=1 W  enable_faults=ee.enum.enable.no  fault_action=simscape.enum.assert.action.none  Cscale_faulted=100  R_faulted=1e-3 Ohm  G_faulted=0 1/Ohm  tau_fault=1e-3 s  fault_trigger=ee.enum.faults.faultTrigger.temporal  t_fault=1 s  max_permissible_voltage_range=[-100, 100] V  t_fail_on_voltage=1 s  i_specify=off  i_priority=None  i=0 A  i_nominal_specify=off  i_nominal_unit=A  i_nominal_value=1  v_specify=off  v_priority=None  v=0 V  v_nominal_specify=off  v_nominal_unit=V  v_nominal_value=1  vc_specify=off  vc_priority=High  vc=0 V  vc_nominal_specify=off  vc_nominal_unit=V  vc_nominal_value=1
  Inverter Efficiency Loss : ee_lib/Passive/Dynamic Load  load_type=ee.enum.dc_ac.dc  min_supply_voltage=1 V  pow_min=1e-3 W  G_reverse=1e-6 S  deltaV=1e-3 V  f0=60 Hz  Vrms_min=200 V  Pmin=1e-3 W  enable_fault=simscape.enum.onoff.off  fault_action=simscape.enum.assert.action.none  t_fault=1 s  open_conductance=1e-4 S
      settings: InternalSimscapePortConfiguration="{\"Bottom\":[],\"Left\":[{\"id\":\"p\",\"label\":\"+\",\"type\":\"foundation.electrical.electrical\"}],\"Right\":[{\"id\":\"n\",\"label\":\"-\",\"type\":\"foundation.electrical.electrical\"}],\"Top\":[{\"id\":\"P\",\"label\":\"P\",\"type\":\"input\"}]}"
  Inverter Power Efficiency : Gain  Gain=1 - 0.98
  PS-Simulink Converter : nesl_utility/PS-Simulink Converter  PhysicalDomain=network_engine_domain  SubClassName=ps_output  LeftPortType=input  RightPortType=output  PseudoPeriodic=off  Frequencies=[]  VectorFormat=inherit  Unit=inherit  AffineConversion=off
  PS-Simulink Converter1 : nesl_utility/PS-Simulink Converter  PhysicalDomain=network_engine_domain  SubClassName=ps_output  LeftPortType=input  RightPortType=output  PseudoPeriodic=off  Frequencies=[]  VectorFormat=inherit  Unit=inherit  AffineConversion=off
  Product : Product
  Simulink-PS Converter : nesl_utility/Simulink-PS Converter  PhysicalDomain=network_engine_domain  SubClassName=ps_input  LeftPortType=input  RightPortType=output  PseudoPeriodic=off  Frequencies=[]  NoiseDistribution=none  NoiseParameters=[]  Unit=1  AffineConversion=off  FilteringAndDerivatives=provide  SimscapeFilterOrder=1  InputFilterTimeConstant=0.001  UdotUserProvided=0
  Simulink-PS Converter1 : nesl_utility/Simulink-PS Converter  PhysicalDomain=network_engine_domain  SubClassName=ps_input  LeftPortType=input  RightPortType=output  PseudoPeriodic=off  Frequencies=[]  NoiseDistribution=none  NoiseParameters=[]  Unit=1  AffineConversion=off  FilteringAndDerivatives=provide  SimscapeFilterOrder=1  InputFilterTimeConstant=0.001  UdotUserProvided=0
  Voltage Sensor : fl_lib/Electrical/Electrical Sensors/Voltage Sensor
  TS + : PMIOPort  Side=Left
  TS - : PMIOPort  Port=2  Side=Right
  Battery Limited Power (W) : Outport
  wires:
  Requested Power (W)/1 -> Inverter Power Efficiency/1, Simulink-PS Converter/1
  PS-Simulink Converter1/1 -> Product/1
  PS-Simulink Converter/1 -> Product/2
  Inverter Power Efficiency/1 -> Simulink-PS Converter1/1
  Product/1 -> Battery Limited Power (W)/1
  connections:
  Inverter Efficiency Loss/RConn1 -- Dynamic Load/RConn1 -- TS -/RConn1 -- Voltage Sensor/RConn2 -- Input Capacitor/RConn1
  Current Sensor/LConn1 -- Inverter Efficiency Loss/LConn1 -- TS +/RConn1 -- Voltage Sensor/LConn1 -- Input Capacitor/LConn1
  Simulink-PS Converter/RConn1 -- Dynamic Load/LConn2
  Voltage Sensor/RConn1 -- PS-Simulink Converter/LConn1
  Current Sensor/RConn2 -- Dynamic Load/LConn1
  PS-Simulink Converter1/LConn1 -- Current Sensor/RConn1
  Simulink-PS Converter1/RConn1 -- Inverter Efficiency Loss/LConn2

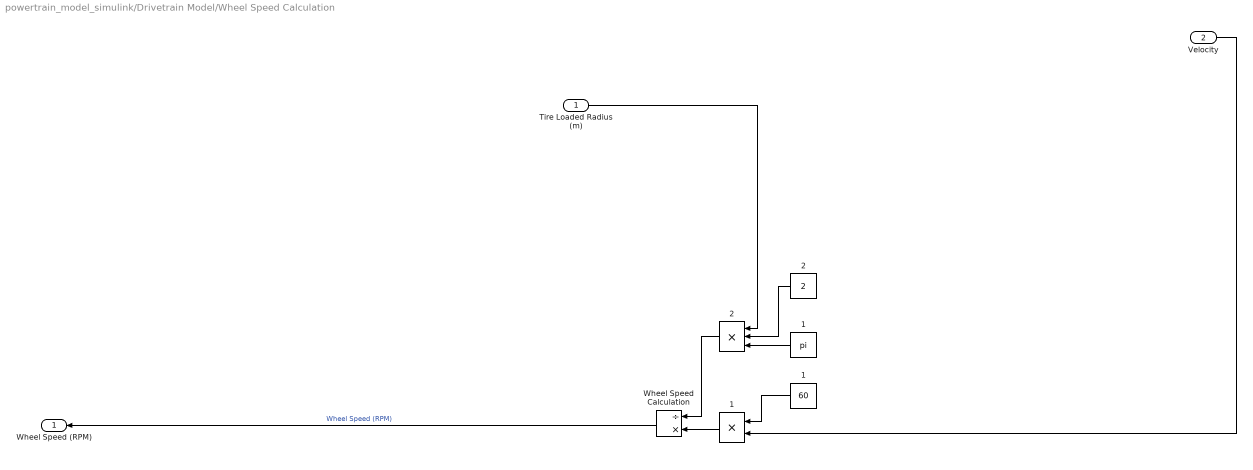
== system powertrain_model_simulink/Drivetrain Model/Wheel Speed Calculation ==
  Tire Loaded Radius (m) : Inport
  Velocity : Inport  Port=2
  "  1" : Product
  "  2" : Product  Inputs=3
  " 1" : Constant  Value=60
  1 : Constant  Value=pi
  2 : Constant  Value=2
  Wheel Speed Calculation : Product  Inputs=/*
  Wheel Speed (RPM) : Outport
  wires:
  Tire Loaded Radius (m)/1 -> "  2"/1
  Velocity/1 -> "  1"/2
  " 1"/1 -> "  1"/1
  "  2"/1 -> Wheel Speed Calculation/1
  1/1 -> "  2"/3
  "  1"/1 -> Wheel Speed Calculation/2
  Wheel Speed Calculation/1 -> Wheel Speed (RPM)/1  "Wheel Speed (RPM)"
  2/1 -> "  2"/2

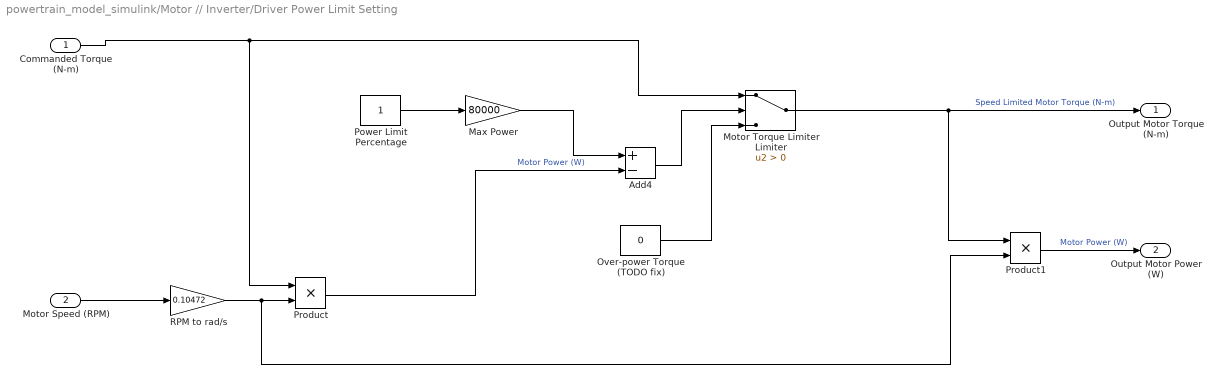
== system powertrain_model_simulink/Motor // Inverter/Driver Power Limit Setting ==
  Commanded Torque (N-m) : Inport
  Motor Speed (RPM) : Inport  Port=2
  Add4 : Sum  Inputs=+-
  Max Power : Gain  Gain=80000
  Motor Torque Limiter Limiter : Switch  Criteria=u2 > Threshold  SaturateOnIntegerOverflow=off  InputSameDT=off
  Over-power Torque (TODO fix) : Constant  Value=0
  Power Limit Percentage : Constant
  Product : Product
  Product1 : Product
  RPM to rad/s : Gain  Gain=0.10472
  Output Motor Torque (N-m) : Outport
  Output Motor Power (W) : Outport  Port=2
  wires:
  Add4/1 -> Motor Torque Limiter Limiter/2
  Commanded Torque (N-m)/1 -> Motor Torque Limiter Limiter/1, Product/1
  Motor Torque Limiter Limiter/1 -> Product1/1, Output Motor Torque (N-m)/1  "Speed Limited Motor Torque (N-m)"
  Over-power Torque (TODO fix)/1 -> Motor Torque Limiter Limiter/3
  Motor Speed (RPM)/1 -> RPM to rad/s/1
  Power Limit Percentage/1 -> Max Power/1
  Product/1 -> Add4/2  "Motor Power (W)"
  Max Power/1 -> Add4/1
  RPM to rad/s/1 -> Product1/2, Product/2
  Product1/1 -> Output Motor Power (W)/1  "Motor Power (W)"

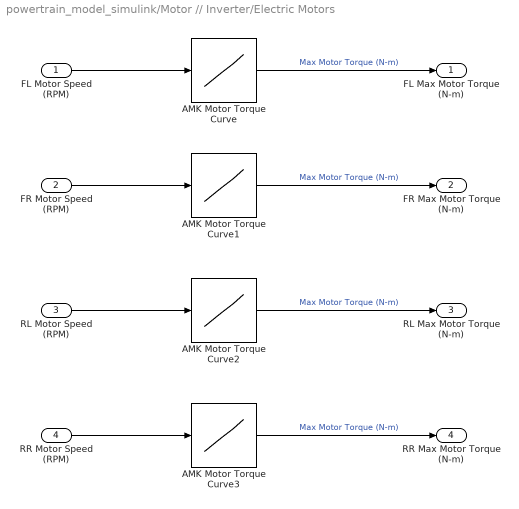
== system powertrain_model_simulink/Motor // Inverter/Electric Motors ==
  FL Motor Speed (RPM) : Inport
  FR Motor Speed (RPM) : Inport  Port=2
  RL Motor Speed (RPM) : Inport  Port=3
  RR Motor Speed (RPM) : Inport  Port=4
  AMK Motor Torque Curve{,1..3} (4 alike) : Lookup_n-D  NumberOfTableDimensions=1  BreakpointsForDimension1=[0;28.3870968;1447.74194;3179.35484;4740.64516;7267.09677;9055.48387;10872.2581;12178.0645;13029.6774;13994.8387;14846.4516;15612.9032;16095.4839;16805.1613;17571.6129;18423.2258;19274.8387;19785.8065;19984.5161]  Table=[21.31;21.3068182;21.3068182;21.3068182;21.3068182;21.3068182;21.3068182;21.3068182;21.3068182;21.3068182;21.3068182;21.3068182;21.3068182;20.9659091;19.9431818;18.5795455;17.0454545;15.3409091;14.1477273;13.6363636]  InternalRulePriority=Speed  RndMeth=Simplest
  FL Max Motor Torque (N-m) : Outport
  FR Max Motor Torque (N-m) : Outport  Port=2
  RL Max Motor Torque (N-m) : Outport  Port=3
  RR Max Motor Torque (N-m) : Outport  Port=4
  wires:
  AMK Motor Torque Curve/1 -> FL Max Motor Torque (N-m)/1  "Max Motor Torque (N-m)"
  FL Motor Speed (RPM)/1 -> AMK Motor Torque Curve/1
  FR Motor Speed (RPM)/1 -> AMK Motor Torque Curve1/1
  AMK Motor Torque Curve1/1 -> FR Max Motor Torque (N-m)/1  "Max Motor Torque (N-m)"
  RL Motor Speed (RPM)/1 -> AMK Motor Torque Curve2/1
  AMK Motor Torque Curve2/1 -> RL Max Motor Torque (N-m)/1  "Max Motor Torque (N-m)"
  RR Motor Speed (RPM)/1 -> AMK Motor Torque Curve3/1
  AMK Motor Torque Curve3/1 -> RR Max Motor Torque (N-m)/1  "Max Motor Torque (N-m)"

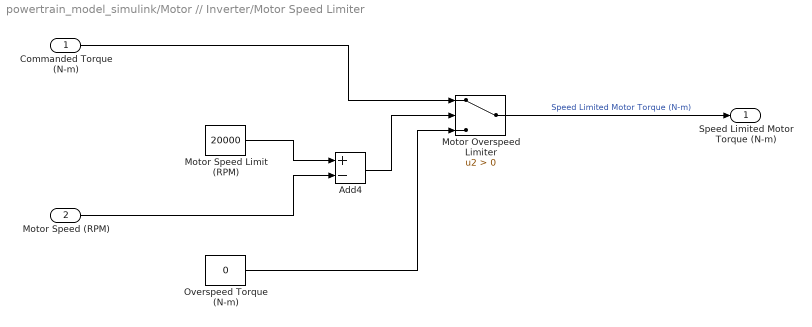
== system powertrain_model_simulink/Motor // Inverter/Motor Speed Limiter ==
  Commanded Torque (N-m) : Inport
  Motor Speed (RPM) : Inport  Port=2
  Add4 : Sum  Inputs=+-
  Motor Overspeed Limiter : Switch  Criteria=u2 > Threshold  SaturateOnIntegerOverflow=off  InputSameDT=off
  Motor Speed Limit (RPM) : Constant  Value=20000
  Overspeed Torque (N-m) : Constant  Value=0
  Speed Limited Motor Torque (N-m) : Outport
  wires:
  Motor Speed (RPM)/1 -> Add4/2
  Add4/1 -> Motor Overspeed Limiter/2
  Commanded Torque (N-m)/1 -> Motor Overspeed Limiter/1
  Motor Speed Limit (RPM)/1 -> Add4/1
  Motor Overspeed Limiter/1 -> Speed Limited Motor Torque (N-m)/1  "Speed Limited Motor Torque (N-m)"
  Overspeed Torque (N-m)/1 -> Motor Overspeed Limiter/3
